simulink model "L3_4_plot_results"  (R2025b)
settings: Solver=VariableStepAuto  StartTime=0.0  StopTime=5  MaxStep=0.01  RelTol=1e-3
settings Model: Creator=kimsteph  LastModifiedBy=kimsteph

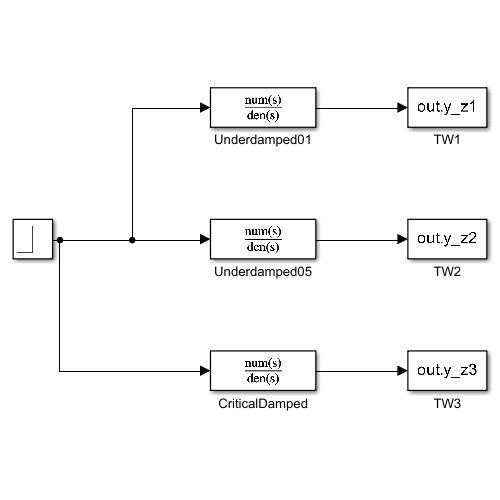
[thumbnail: Simulink's stored preview of the top-level diagram]
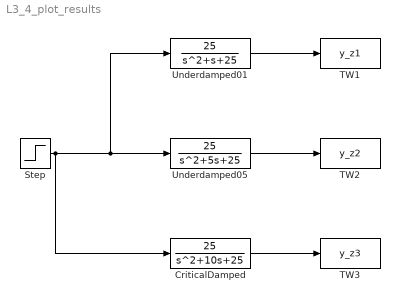
== system L3_4_plot_results ==
  CriticalDamped : TransferFcn  Numerator=25  Denominator=[1 10 25]
  Step : Step  Time=0  SampleTime=0
  TW1 : ToWorkspace  VariableName=y_z1  SaveFormat=Timeseries  SampleTime=-1
  TW2 : ToWorkspace  VariableName=y_z2  SaveFormat=Timeseries  SampleTime=-1
  TW3 : ToWorkspace  VariableName=y_z3  SaveFormat=Timeseries  SampleTime=-1
  Underdamped01 : TransferFcn  Numerator=25  Denominator=[1 1 25]
  Underdamped05 : TransferFcn  Numerator=25  Denominator=[1 5 25]
  wires:
  Step/1 -> Underdamped01/1, Underdamped05/1, CriticalDamped/1
  Underdamped01/1 -> TW1/1
  Underdamped05/1 -> TW2/1
  CriticalDamped/1 -> TW3/1
